simulink model "QuadcopterLinearZero"  (R2020a)
settings: Solver=ode4  StartTime=0.0  StopTime=10.0  FixedStep=0.1  RelTol=1e-3
undefined symbols (not defined in the file): A1, A3, B1, B3, C2
settings Model: Creator=Ali  LastModifiedBy=Ali

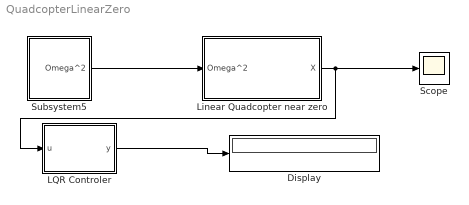
== system QuadcopterLinearZero ==
  Display : Display
  LQR Controler : MATLAB Function  TreatAsAtomicUnit=on
  Linear Quadcopter near zero : Subsystem
      mask Display: image('E:\University\bachelor-thesis\Code\Simulink\Quadcopter\drone_PNG203.png'); % Use "Edit Image" on toolstrip to change.
  Scope : Scope
  Subsystem5 : Subsystem
  wires:
  Linear Quadcopter near zero/1(X) -> LQR Controler/1(u), Scope/1
  LQR Controler/1(y) -> Display/1
  Subsystem5/1(Omega^2) -> Linear Quadcopter near zero/1(Omega^2)

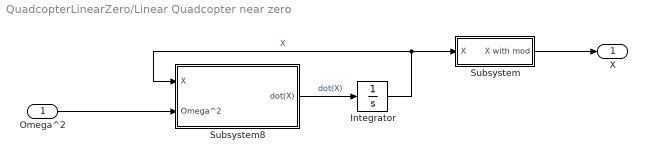
== system QuadcopterLinearZero/Linear Quadcopter near zero ==
  Omega^2 : Inport
  Integrator : Integrator
  Subsystem : Subsystem
  Subsystem8 : Subsystem
  X : Outport
  wires:
  Integrator/1 -> Subsystem8/1(X), Subsystem/1(X)  "X"
  Subsystem8/1(dot(X)) -> Integrator/1  "dot(X)"
  Omega^2/1 -> Subsystem8/2(Omega^2)
  Subsystem/1(X with mod) -> X/1

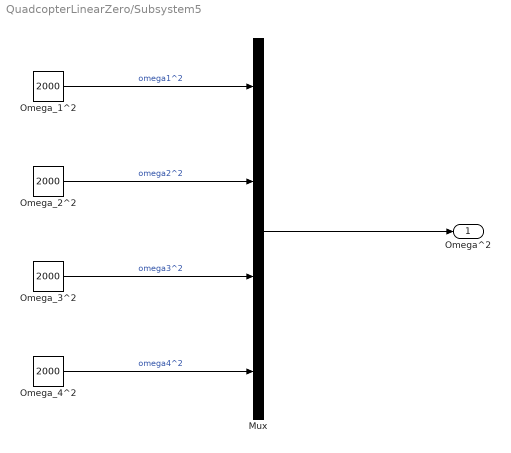
== system QuadcopterLinearZero/Subsystem5 ==
  Mux : Mux
  Omega_1^2 : Constant  Value=2000
  Omega_2^2 : Constant  Value=2000
  Omega_3^2 : Constant  Value=2000
  Omega_4^2 : Constant  Value=2000
  Omega^2 : Outport
  wires:
  Omega_2^2/1 -> Mux/2  "omega2^2"
  Omega_3^2/1 -> Mux/3  "omega3^2"
  Omega_4^2/1 -> Mux/4  "omega4^2"
  Omega_1^2/1 -> Mux/1  "omega1^2"
  Mux/1 -> Omega^2/1

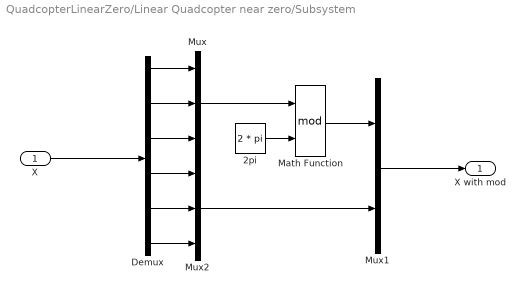
== system QuadcopterLinearZero/Linear Quadcopter near zero/Subsystem ==
  X : Inport
  2pi : Constant  Value=2 * pi
  Demux : Demux  Outputs=6
  Math Function : Math  Operator=mod  SaturateOnIntegerOverflow=on
  Mux : Mux  Inputs=3
  Mux1 : Mux  Inputs=2
  Mux2 : Mux  Inputs=3
  X with mod : Outport
  wires:
  X/1 -> Demux/1
  Demux/1 -> Mux/1
  Demux/2 -> Mux/2
  Demux/3 -> Mux/3
  Demux/4 -> Mux2/1
  Demux/5 -> Mux2/2
  Demux/6 -> Mux2/3
  Math Function/1 -> Mux1/1
  Mux2/1 -> Mux1/2
  Mux1/1 -> X with mod/1
  2pi/1 -> Math Function/2
  Mux/1 -> Math Function/1

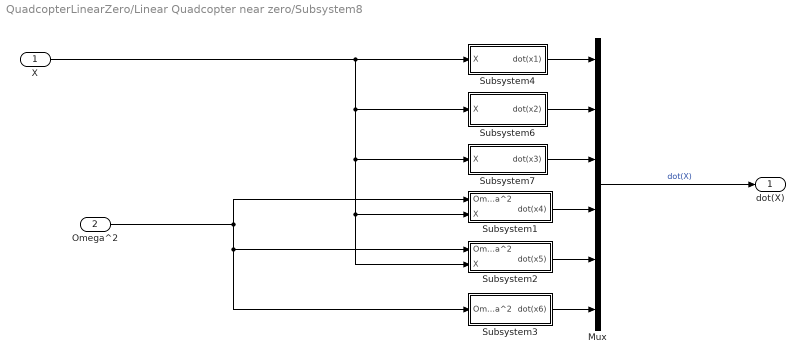
== system QuadcopterLinearZero/Linear Quadcopter near zero/Subsystem8 ==
  X : Inport
  Omega^2 : Inport  Port=2
  Mux : Mux  Inputs=6
  Subsystem1 : Subsystem
  Subsystem2 : Subsystem
  Subsystem3 : Subsystem
  Subsystem4 : Subsystem
  Subsystem6 : Subsystem
  Subsystem7 : Subsystem
  dot(X) : Outport
  wires:
  Omega^2/1 -> Subsystem2/1(Omega^2), Subsystem3/1(Omega^2), Subsystem1/1(Omega^2)
  Subsystem3/1(dot(x6)) -> Mux/6
  Subsystem7/1(dot(x3)) -> Mux/3
  Subsystem1/1(dot(x4)) -> Mux/4
  Subsystem6/1(dot(x2)) -> Mux/2
  X/1 -> Subsystem2/2(X), Subsystem1/2(X), Subsystem7/1(X), Subsystem6/1(X), Subsystem4/1(X)
  Subsystem2/1(dot(x5)) -> Mux/5
  Subsystem4/1(dot(x1)) -> Mux/1
  Mux/1 -> dot(X)/1  "dot(X)"

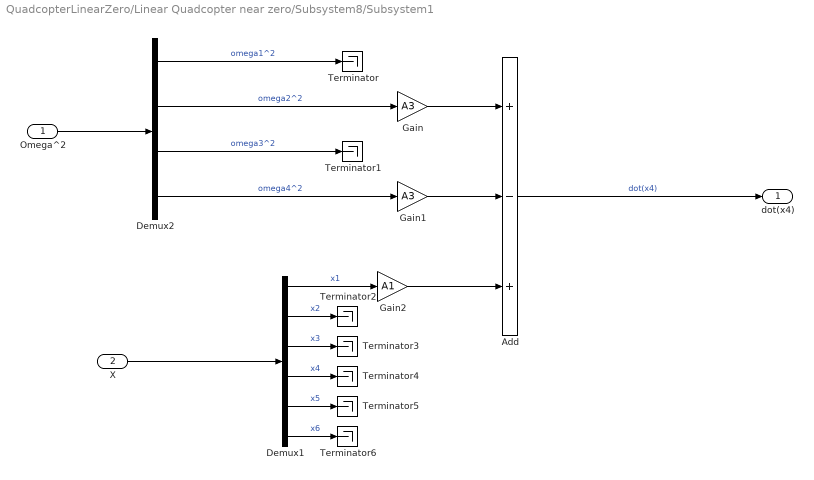
== system QuadcopterLinearZero/Linear Quadcopter near zero/Subsystem8/Subsystem1 ==
  Omega^2 : Inport
  X : Inport  Port=2
  Add : Sum  Inputs=+-+
  Demux1 : Demux  Outputs=6
  Demux2 : Demux
  Gain : Gain  Gain=A3
  Gain1 : Gain  Gain=A3
  Gain2 : Gain  Gain=A1
  Terminator{,1..6} (7 alike) : Terminator
  dot(x4) : Outport
  wires:
  Gain2/1 -> Add/3
  Gain1/1 -> Add/2
  Add/1 -> dot(x4)/1  "dot(x4)"
  Gain/1 -> Add/1
  Demux2/4 -> Gain1/1  "omega4^2"
  Demux2/2 -> Gain/1  "omega2^2"
  Demux2/3 -> Terminator1/1  "omega3^2"
  Demux2/1 -> Terminator/1  "omega1^2"
  Omega^2/1 -> Demux2/1
  Demux1/5 -> Terminator5/1  "x5"
  Demux1/2 -> Terminator2/1  "x2"
  Demux1/3 -> Terminator3/1  "x3"
  Demux1/1 -> Gain2/1  "x1"
  Demux1/4 -> Terminator4/1  "x4"
  X/1 -> Demux1/1
  Demux1/6 -> Terminator6/1  "x6"

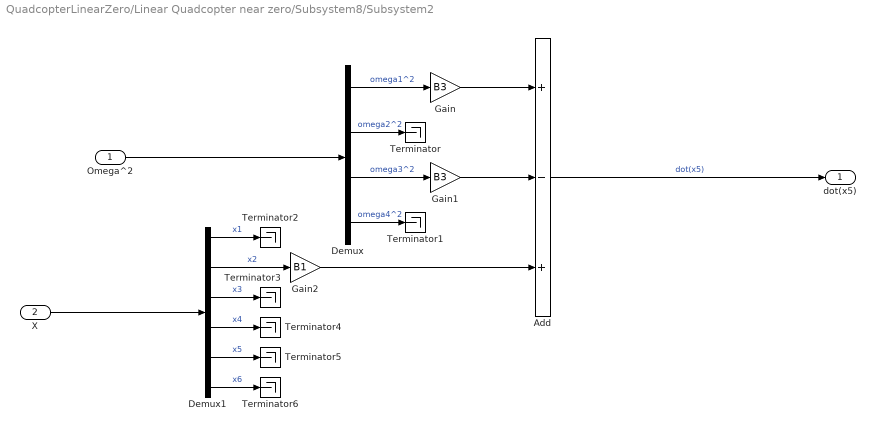
== system QuadcopterLinearZero/Linear Quadcopter near zero/Subsystem8/Subsystem2 ==
  Omega^2 : Inport
  X : Inport  Port=2
  Add : Sum  Inputs=+-+
  Demux : Demux
  Demux1 : Demux  Outputs=6
  Gain : Gain  Gain=B3
  Gain1 : Gain  Gain=B3
  Gain2 : Gain  Gain=B1
  Terminator{,1..6} (7 alike) : Terminator
  dot(x5) : Outport
  wires:
  Gain2/1 -> Add/3
  Gain1/1 -> Add/2
  Add/1 -> dot(x5)/1  "dot(x5)"
  Gain/1 -> Add/1
  Omega^2/1 -> Demux/1
  Demux/2 -> Terminator/1  "omega2^2"
  Demux/4 -> Terminator1/1  "omega4^2"
  Demux/1 -> Gain/1  "omega1^2"
  Demux/3 -> Gain1/1  "omega3^2"
  Demux1/5 -> Terminator5/1  "x5"
  Demux1/2 -> Gain2/1  "x2"
  Demux1/3 -> Terminator3/1  "x3"
  Demux1/1 -> Terminator2/1  "x1"
  Demux1/4 -> Terminator4/1  "x4"
  X/1 -> Demux1/1
  Demux1/6 -> Terminator6/1  "x6"

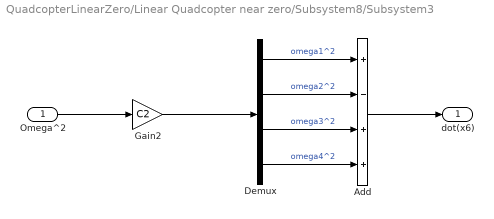
== system QuadcopterLinearZero/Linear Quadcopter near zero/Subsystem8/Subsystem3 ==
  Omega^2 : Inport
  Add : Sum  Inputs=+-++
  Demux : Demux
  Gain2 : Gain  Gain=C2
  dot(x6) : Outport
  wires:
  Omega^2/1 -> Gain2/1
  Gain2/1 -> Demux/1
  Demux/1 -> Add/1  "omega1^2"
  Demux/2 -> Add/2  "omega2^2"
  Demux/3 -> Add/3  "omega3^2"
  Demux/4 -> Add/4  "omega4^2"
  Add/1 -> dot(x6)/1

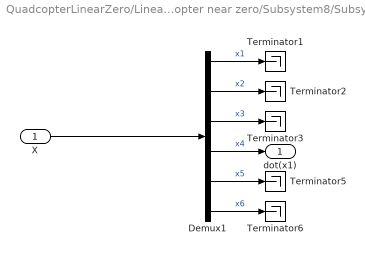
== system QuadcopterLinearZero/Linear Quadcopter near zero/Subsystem8/Subsystem4 ==
  X : Inport
  Demux1 : Demux  Outputs=6
  Terminator{1..3,5..6} (5 alike) : Terminator
  dot(x1) : Outport
  wires:
  Demux1/4 -> dot(x1)/1  "x4"
  X/1 -> Demux1/1
  Demux1/6 -> Terminator6/1  "x6"
  Demux1/5 -> Terminator5/1  "x5"
  Demux1/3 -> Terminator3/1  "x3"
  Demux1/2 -> Terminator2/1  "x2"
  Demux1/1 -> Terminator1/1  "x1"

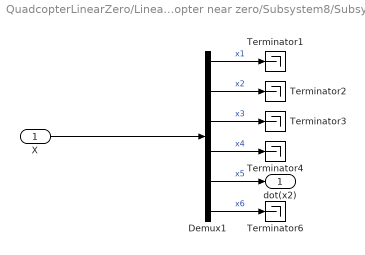
== system QuadcopterLinearZero/Linear Quadcopter near zero/Subsystem8/Subsystem6 ==
  X : Inport
  Demux1 : Demux  Outputs=6
  Terminator{1..4,6} (5 alike) : Terminator
  dot(x2) : Outport
  wires:
  Demux1/4 -> Terminator4/1  "x4"
  X/1 -> Demux1/1
  Demux1/6 -> Terminator6/1  "x6"
  Demux1/5 -> dot(x2)/1  "x5"
  Demux1/3 -> Terminator3/1  "x3"
  Demux1/2 -> Terminator2/1  "x2"
  Demux1/1 -> Terminator1/1  "x1"

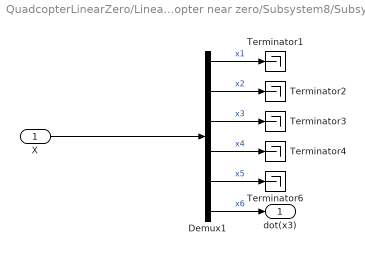
== system QuadcopterLinearZero/Linear Quadcopter near zero/Subsystem8/Subsystem7 ==
  X : Inport
  Demux1 : Demux  Outputs=6
  Terminator{1..4,6} (5 alike) : Terminator
  dot(x3) : Outport
  wires:
  Demux1/4 -> Terminator4/1  "x4"
  X/1 -> Demux1/1
  Demux1/6 -> dot(x3)/1  "x6"
  Demux1/5 -> Terminator6/1  "x5"
  Demux1/3 -> Terminator3/1  "x3"
  Demux1/2 -> Terminator2/1  "x2"
  Demux1/1 -> Terminator1/1  "x1"

== matlab function QuadcopterLinearZero/LQR Controler ==
  data: u input; y output
function y = fcn(u)
% Distance between rotor center to quad center (m)
d_cg = 0.295;
% Distance between D point to quad center (m)
h_cg = 0.0078;
% Thrust factor (non dimensional)
b = 1.10794e-5;
% Rotor torque drag factor (non dimensional)
d = 3.2e-6;
% Total mass (kg)
m_tot = 1.774;
% Quad Moment of inertia respect to axix X Body (kg.m^2)
J_xx = 0.0297598;
% Quad Moment of inertia respect to axix Y Body (kg.m^2)
J_yy = 0.0298565;
% Quad Moment of inertia respect to axix Y Body (kg.m^2)
J_zz = 0.058510;
% Quad blade Moment (kg.m^2)
%J_R = 4.439e-5;
% Mass on X axis bearing (kg)
%m1 = 1.272;
% Mass on Y axis bearing (kg)
%m2 = 1.074;
% Mass on Z axis bearing (kg)
%m3 = 1.693;
% Bearing radius in X axix (m)
%r_x = 0.01;
% Bearing radius in Y axix (m)
%r_y = 0.01;
% Bearing radius in Z axix (m)
%r_z = 0.025;
% Static bearing friction (non dimensional)
%miu_s = 0.003;
% Dynamic bearing friction (non dimensional)
%miu_k = 0.002;
% Motor constant (non dimensional)
%tau = 0.15;
% Delay of motor (sec)
%T_d = 0.02;
% Gravity force (m/s^2)
g = 9.81;
% A Constants
A1 = (h_cg * g * m_tot) / (m_tot * h_cg^2 + J_xx);
%A2 = (2*m_tot * h_cg^2 + J_yy -J_zz) / (m_tot * h_cg^2 + J_xx);
A3 = (b * d_cg) / (m_tot * h_cg^2 + J_xx);
%A4 = (J_R) / (m_tot * h_cg^2 + J_xx);
%A5 = (m1 * g * miu_k * r_x) / (m_tot * h_cg^2 + J_xx);
% B Constants
B1 = (h_cg * g * m_tot) / (m_tot * h_cg^2 + J_yy);
%B2 = (-2*m_tot * h_cg^2 - J_xx + J_zz) / (m_tot * h_cg^2 + J_yy);
B3 = (b * d_cg) / (m_tot * h_cg^2 + J_yy);
%B4 = (-J_R) / (m_tot * h_cg^2 + J_yy);
%B5 = (m2 * g * miu_k * r_y) / (m_tot * h_cg^2 + J_yy);
% C Constants
%C1 = (J_xx - J_yy) / (J_zz);
C2 = (d) / (J_zz);
%C3 = (m3 * g * miu_k * r_z) / (J_zz);
A = [0  0  0 1 0 0  ;
     0  0  0 0 1 0  ;
     0  0  0 0 0 1  ;
     A1 0  0 0 0 0  ;
     0  B1 0 0 0 0  ;
     0  0  0 0 0 0] ;
B = [0   0   0   0  ;
     0   0   0   0  ;
     0   0   0   0  ;
     0   A3  0  -A3 ;
     B3  0  -B3  0  ;
     C2 -C2  C2  C2];
%% test %%
%%% Quad in zero LQR solver %%%
%QuadSpaceState;
% Weight Matrix %
%syms Q11 Q22 Q33 Q44 Q55 Q66
Q = [1 0   0   0   0   0   ;
     0   1 0   0   0   0   ;
     0   0   1 0   0   0   ;
     0   0   0   1 0   0   ;
     0   0   0   0   1 0   ;
     0   0   0   0   0  1];
R = [1 0   0   0   ;
     0   1 0   0   ;
     0   0   1 0   ;
     0   0   0   1];
% Riccati Solver %
% algebraic_riccati = K * A + A' * K - K * B * R^-1 * B' * K + Q
coder.extrinsic('icare');
K = zeros(4, 6);
[X, K, Y] = icare(A, B, Q, R);
y = R^-1 * B' * K * u;
